simulink model "s_heli3d_fuzzy"  (R2023a)
settings: Solver=ode1  StartTime=0.0  StopTime=60  FixedStep=0.002  RelTol=1e-3  EnableMultiTasking=on
values from neighbouring files (symbols this model uses):
  A = sys.A    [read_model.m]
  B = sys.B    [read_model.m]
  CMD_RATE_LIMIT = 45.0 * pi / 180    (= 0.785398163397)    [setup_lab_heli_3d.m]
  K_AMP = 3    [setup_lab_heli_3d.m]
  VMAX_AMP = 24    [setup_lab_heli_3d.m]
  VMAX_DAC = 10    [setup_lab_heli_3d.m]
libraries: simulink_extras x6, statsLibrary x4
settings Model: ExtModeTrigDuration=5000  Creator=MLevis  LastModifiedBy=hackbrian
settings SolverCC: AlgebraicLoopSolver=TrustRegion  PositivePriorityOrder=on
settings DataIOCC: LimitDataPoints=on  SaveFormat=Array  SignalLoggingSaveFormat=ModelDataLogs  ReturnWorkspaceOutputs=off
settings OptimizationCC: BooleanDataType=off  OptimizeBlockIOStorage=off  BufferReuse=off  ExpressionFolding=off  ExpressionDepthLimit=2147483647  LocalBlockOutputs=off  InitFltsAndDblsToZero=on  LifeSpan=inf
settings DebuggingCC: SaveWithParameterizedLinksMsg=none  UnderspecifiedInitializationDetection=Classic  MergeDetectMultiDrivingBlocksExec=none  SignalResolutionControl=TryResolveAllWithWarning  SolverPrmCheckMsg=warning  MultiTaskDSMMsg=warning  MultiTaskCondExecSysMsg=none  FcnCallInpInsideContextMsg=warning  UnconnectedInputMsg=warning  UnconnectedOutputMsg=warning  UnconnectedLineMsg=warning  StateNameClashWarn=warning  SFUnexpectedBacktrackingDiag=warning  SFNoUnconditionalDefaultTransitionDiag=warning  SFExecutionAtInitializationDiag=none  ArithmeticOperatorsInVariantConditions=warning
settings HardwareCC: ProdBitPerPointer=32  ProdBitPerSizeT=32  ProdBitPerPtrDiffT=32  ProdLargestAtomicFloat=None  ProdIntDivRoundTo=Undefined  ProdEndianess=Unspecified  ProdWordSize=32  ProdHWDeviceType=32-bit Generic
settings ModelReferenceCC: PropagateSignalLabelsOutOfModel=off
settings RTWCC: Description=QUARC Win32 Target  SystemTargetFile=quarc_windows.tlc  TemplateMakefile=quarc_default_tmf
settings CodeAppCC: StateflowObjectComments=on
settings STFCustomTargetCC: TargetFcnLib=ansi_tfl_tmw.mat  TargetPreCompLibLocation=C:\DOCUME~1\ALLUSE~1\APPLIC~1\QUARC\lib\2007a\windows\release  TargetLangStandard=C89/C90 (ANSI)  ConcurrentExecutionCompliant=off  CPPClassGenCompliant=on  UseToolchainInfoCompliant=off  SystemTargetFile=quarc_windows.tlc
settings GRTTargetCC: TargetFcnLib=ansi_tfl_tmw.mat  TargetPreCompLibLocation=C:\DOCUME~1\ALLUSE~1\APPLIC~1\QUARC\lib\2007a\windows\release  TargetLangStandard=C89/C90 (ANSI)  ParMdlRefBuildCompliant=off  CompOptLevelCompliant=off  ConcurrentExecutionCompliant=off  CombineOutputUpdateFcns=off  MatFileLogging=off  GRTInterface=on  UseToolchainInfoCompliant=off  ExtMode=on  ExtModeMexFile=quarc_comm
settings ConfigComp: CovMetricSettings=dw  CovSaveCumulativeToWorkspaceVar=on  CovSaveSingleToWorkspaceVar=on

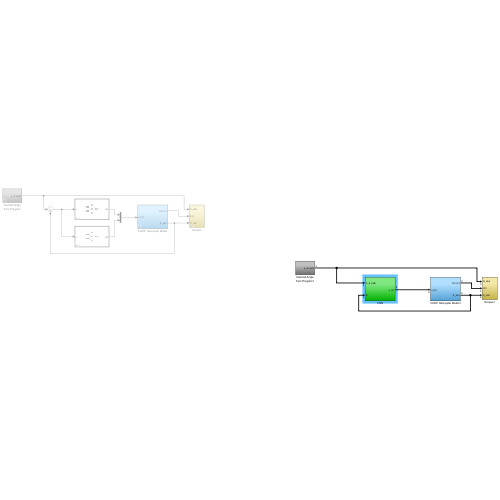
[thumbnail: Simulink's stored preview of the top-level diagram]
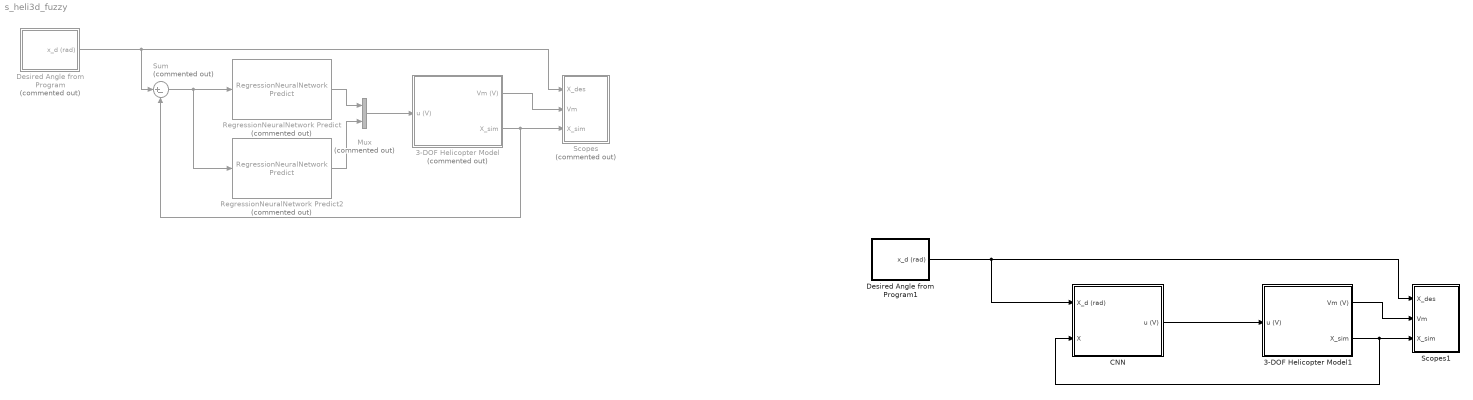
== system s_heli3d_fuzzy ==
  3-DOF Helicopter Model : Subsystem  Commented=on
  3-DOF Helicopter Model1 : Subsystem
  CNN : Subsystem  AncestorBlock=heli_2d_lib/2DOF HELI: FF+LQR+I Controller
      settings: LibrarySourceBlock=|
      | heli_2d_lib/2DOF HELI:
      | FF+LQR+I Controller
  Desired Angle from Program : Subsystem  Commented=on
  Desired Angle from Program1 : Subsystem
  Mux : Mux  Commented=on  Inputs=2
  RegressionNeuralNetwork Predict : statsLibrary/Regression/RegressionNeuralNetwork Predict  Commented=on  TrainedLearner=Mdl_voltage1  OutMin=[]  OutMax=[]  OutputLayerOutMin=[]  OutputLayerOutMax=[]  OutputLayerAdditionOutMin=[]  OutputLayerAdditionOutMax=[]  LayerSelector=Layer 1  Layer1OutMin=[]  Layer1OutMax=[]  Layer1AdditionOutMin=[]  Layer1AdditionOutMax=[]  Layer2OutMin=[]  Layer2OutMax=[]  Layer2AdditionOutMin=[]  Layer2AdditionOutMax=[]  Layer3OutMin=[]  Layer3OutMax=[]  Layer3AdditionOutMin=[]  Layer3AdditionOutMax=[]  Layer4OutMin=[]  Layer4OutMax=[]  Layer4AdditionOutMin=[]  Layer4AdditionOutMax=[]  Layer5OutMin=[]  Layer5OutMax=[]  Layer5AdditionOutMin=[]  Layer5AdditionOutMax=[]  Layer6OutMin=[]  Layer6OutMax=[]  Layer6AdditionOutMin=[]  Layer6AdditionOutMax=[]  Layer7OutMin=[]  Layer7OutMax=[]  Layer7AdditionOutMin=[]  Layer7AdditionOutMax=[]  Layer8OutMin=[]  Layer8OutMax=[]  Layer8AdditionOutMin=[]  Layer8AdditionOutMax=[]  Layer9OutMin=[]  Layer9OutMax=[]  Layer9AdditionOutMin=[]  Layer9AdditionOutMax=[]  Layer10OutMin=[]  Layer10OutMax=[]  Layer10AdditionOutMin=[]  Layer10AdditionOutMax=[]  Layer11OutMin=[]  Layer11OutMax=[]  Layer11AdditionOutMin=[]  Layer11AdditionOutMax=[]  StandardizedInputOutMin=[]  StandardizedInputOutMax=[]  NumHiddenLayers=1
  RegressionNeuralNetwork Predict2 : statsLibrary/Regression/RegressionNeuralNetwork Predict  Commented=on  TrainedLearner=Mdl_voltage2  OutMin=[]  OutMax=[]  OutputLayerOutMin=[]  OutputLayerOutMax=[]  OutputLayerAdditionOutMin=[]  OutputLayerAdditionOutMax=[]  LayerSelector=Layer 1  Layer1OutMin=[]  Layer1OutMax=[]  Layer1AdditionOutMin=[]  Layer1AdditionOutMax=[]  Layer2OutMin=[]  Layer2OutMax=[]  Layer2AdditionOutMin=[]  Layer2AdditionOutMax=[]  Layer3OutMin=[]  Layer3OutMax=[]  Layer3AdditionOutMin=[]  Layer3AdditionOutMax=[]  Layer4OutMin=[]  Layer4OutMax=[]  Layer4AdditionOutMin=[]  Layer4AdditionOutMax=[]  Layer5OutMin=[]  Layer5OutMax=[]  Layer5AdditionOutMin=[]  Layer5AdditionOutMax=[]  Layer6OutMin=[]  Layer6OutMax=[]  Layer6AdditionOutMin=[]  Layer6AdditionOutMax=[]  Layer7OutMin=[]  Layer7OutMax=[]  Layer7AdditionOutMin=[]  Layer7AdditionOutMax=[]  Layer8OutMin=[]  Layer8OutMax=[]  Layer8AdditionOutMin=[]  Layer8AdditionOutMax=[]  Layer9OutMin=[]  Layer9OutMax=[]  Layer9AdditionOutMin=[]  Layer9AdditionOutMax=[]  Layer10OutMin=[]  Layer10OutMax=[]  Layer10AdditionOutMin=[]  Layer10AdditionOutMax=[]  Layer11OutMin=[]  Layer11OutMax=[]  Layer11AdditionOutMin=[]  Layer11AdditionOutMax=[]  StandardizedInputOutMin=[]  StandardizedInputOutMax=[]  NumHiddenLayers=1
  Scopes : Subsystem  Commented=on
  Scopes1 : Subsystem
  Sum : Sum  Commented=on  Inputs=|+-
  wires:
  Desired Angle from Program/1(x_d (rad)) -> Sum/1, Scopes/1(X_des)
  3-DOF Helicopter Model/2(X_sim) -> Scopes/3(X_sim), Sum/2
  3-DOF Helicopter Model/1(Vm (V)) -> Scopes/2(Vm)
  Sum/1 -> RegressionNeuralNetwork Predict/1, RegressionNeuralNetwork Predict2/1
  Mux/1 -> 3-DOF Helicopter Model/1(u (V))
  RegressionNeuralNetwork Predict/1 -> Mux/1
  RegressionNeuralNetwork Predict2/1 -> Mux/2
  3-DOF Helicopter Model1/2(X_sim) -> CNN/2(X), Scopes1/3(X_sim)
  Desired Angle from Program1/1(x_d (rad)) -> CNN/1(X_d (rad)), Scopes1/1(X_des)
  3-DOF Helicopter Model1/1(Vm (V)) -> Scopes1/2(Vm)
  CNN/1(u (V)) -> 3-DOF Helicopter Model1/1(u (V))

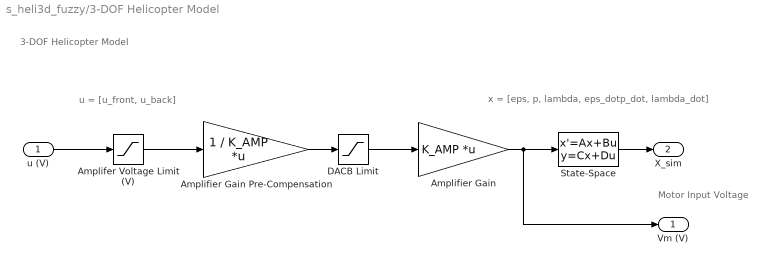
== system s_heli3d_fuzzy/3-DOF Helicopter Model ==
  note: x = [eps, p, lambda, eps_dotp_dot, lambda_dot]
  note: u = [u_front, u_back]
  note: Motor Input Voltage
  note: 3-DOF Helicopter Model
  u (V) : Inport
  Amplifer Voltage Limit (V) : Saturate  UpperLimit=VMAX_AMP  LowerLimit=-VMAX_AMP
  Amplifier Gain : Gain  Gain=K_AMP  Multiplication=Matrix(K*u)  SaturateOnIntegerOverflow=on  OutDataTypeStr=Inherit: Same as input  ParamDataTypeStr=Inherit: Same as input
  Amplifier Gain Pre-Compensation : Gain  Gain=1 / K_AMP  Multiplication=Matrix(K*u)  SaturateOnIntegerOverflow=on  OutDataTypeStr=Inherit: Same as input  ParamDataTypeStr=Inherit: Same as input
  DACB Limit : Saturate  UpperLimit=VMAX_DAC  LowerLimit=-VMAX_DAC
  State-Space : StateSpace  A=A  B=B  C=eye(6,6)  D=zeros(6,2)  InitialCondition=0
  Vm (V) : Outport
  X_sim : Outport  Port=2
  wires:
  u (V)/1 -> Amplifer Voltage Limit (V)/1
  Amplifier Gain/1 -> Vm (V)/1, State-Space/1
  State-Space/1 -> X_sim/1
  Amplifer Voltage Limit (V)/1 -> Amplifier Gain Pre-Compensation/1
  Amplifier Gain Pre-Compensation/1 -> DACB Limit/1
  DACB Limit/1 -> Amplifier Gain/1

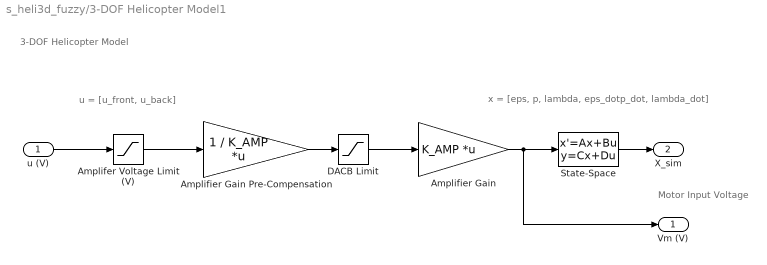
== system s_heli3d_fuzzy/3-DOF Helicopter Model1 ==
  note: x = [eps, p, lambda, eps_dotp_dot, lambda_dot]
  note: u = [u_front, u_back]
  note: Motor Input Voltage
  note: 3-DOF Helicopter Model
  u (V) : Inport
  Amplifer Voltage Limit (V) : Saturate  UpperLimit=VMAX_AMP  LowerLimit=-VMAX_AMP
  Amplifier Gain : Gain  Gain=K_AMP  Multiplication=Matrix(K*u)  SaturateOnIntegerOverflow=on  OutDataTypeStr=Inherit: Same as input  ParamDataTypeStr=Inherit: Same as input
  Amplifier Gain Pre-Compensation : Gain  Gain=1 / K_AMP  Multiplication=Matrix(K*u)  SaturateOnIntegerOverflow=on  OutDataTypeStr=Inherit: Same as input  ParamDataTypeStr=Inherit: Same as input
  DACB Limit : Saturate  UpperLimit=VMAX_DAC  LowerLimit=-VMAX_DAC
  State-Space : StateSpace  A=A  B=B  C=eye(6,6)  D=zeros(6,2)  InitialCondition=0
  Vm (V) : Outport
  X_sim : Outport  Port=2
  wires:
  u (V)/1 -> Amplifer Voltage Limit (V)/1
  Amplifier Gain/1 -> Vm (V)/1, State-Space/1
  State-Space/1 -> X_sim/1
  Amplifer Voltage Limit (V)/1 -> Amplifier Gain Pre-Compensation/1
  Amplifier Gain Pre-Compensation/1 -> DACB Limit/1
  DACB Limit/1 -> Amplifier Gain/1

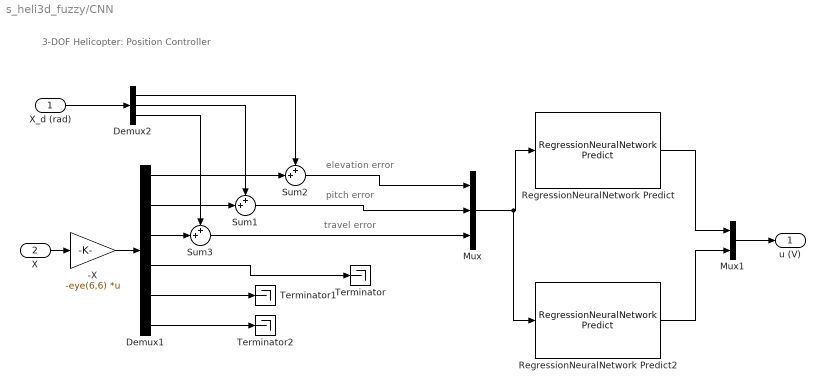
== system s_heli3d_fuzzy/CNN ==
  note: elevation error
  note: pitch error
  note: 3-DOF Helicopter: Position Controller
  note: travel error
  X_d (rad) : Inport
  X : Inport  Port=2
  -X : Gain  Gain=-eye(6,6)  Multiplication=Matrix(K*u)
  Demux1 : Demux  Outputs=6
  Demux2 : Demux  Outputs=3
  Mux : Mux  Inputs=3
  Mux1 : Mux  Inputs=2
  RegressionNeuralNetwork Predict : statsLibrary/Regression/RegressionNeuralNetwork Predict  TrainedLearner=Mdl_voltage1  OutMin=[]  OutMax=[]  OutputLayerOutMin=[]  OutputLayerOutMax=[]  OutputLayerAdditionOutMin=[]  OutputLayerAdditionOutMax=[]  LayerSelector=Layer 1  Layer1OutMin=[]  Layer1OutMax=[]  Layer1AdditionOutMin=[]  Layer1AdditionOutMax=[]  Layer2OutMin=[]  Layer2OutMax=[]  Layer2AdditionOutMin=[]  Layer2AdditionOutMax=[]  Layer3OutMin=[]  Layer3OutMax=[]  Layer3AdditionOutMin=[]  Layer3AdditionOutMax=[]  Layer4OutMin=[]  Layer4OutMax=[]  Layer4AdditionOutMin=[]  Layer4AdditionOutMax=[]  Layer5OutMin=[]  Layer5OutMax=[]  Layer5AdditionOutMin=[]  Layer5AdditionOutMax=[]  Layer6OutMin=[]  Layer6OutMax=[]  Layer6AdditionOutMin=[]  Layer6AdditionOutMax=[]  Layer7OutMin=[]  Layer7OutMax=[]  Layer7AdditionOutMin=[]  Layer7AdditionOutMax=[]  Layer8OutMin=[]  Layer8OutMax=[]  Layer8AdditionOutMin=[]  Layer8AdditionOutMax=[]  Layer9OutMin=[]  Layer9OutMax=[]  Layer9AdditionOutMin=[]  Layer9AdditionOutMax=[]  Layer10OutMin=[]  Layer10OutMax=[]  Layer10AdditionOutMin=[]  Layer10AdditionOutMax=[]  Layer11OutMin=[]  Layer11OutMax=[]  Layer11AdditionOutMin=[]  Layer11AdditionOutMax=[]  StandardizedInputOutMin=[]  StandardizedInputOutMax=[]  NumHiddenLayers=1
  RegressionNeuralNetwork Predict2 : statsLibrary/Regression/RegressionNeuralNetwork Predict  TrainedLearner=Mdl_voltage2  OutMin=[]  OutMax=[]  OutputLayerOutMin=[]  OutputLayerOutMax=[]  OutputLayerAdditionOutMin=[]  OutputLayerAdditionOutMax=[]  LayerSelector=Layer 1  Layer1OutMin=[]  Layer1OutMax=[]  Layer1AdditionOutMin=[]  Layer1AdditionOutMax=[]  Layer2OutMin=[]  Layer2OutMax=[]  Layer2AdditionOutMin=[]  Layer2AdditionOutMax=[]  Layer3OutMin=[]  Layer3OutMax=[]  Layer3AdditionOutMin=[]  Layer3AdditionOutMax=[]  Layer4OutMin=[]  Layer4OutMax=[]  Layer4AdditionOutMin=[]  Layer4AdditionOutMax=[]  Layer5OutMin=[]  Layer5OutMax=[]  Layer5AdditionOutMin=[]  Layer5AdditionOutMax=[]  Layer6OutMin=[]  Layer6OutMax=[]  Layer6AdditionOutMin=[]  Layer6AdditionOutMax=[]  Layer7OutMin=[]  Layer7OutMax=[]  Layer7AdditionOutMin=[]  Layer7AdditionOutMax=[]  Layer8OutMin=[]  Layer8OutMax=[]  Layer8AdditionOutMin=[]  Layer8AdditionOutMax=[]  Layer9OutMin=[]  Layer9OutMax=[]  Layer9AdditionOutMin=[]  Layer9AdditionOutMax=[]  Layer10OutMin=[]  Layer10OutMax=[]  Layer10AdditionOutMin=[]  Layer10AdditionOutMax=[]  Layer11OutMin=[]  Layer11OutMax=[]  Layer11AdditionOutMin=[]  Layer11AdditionOutMax=[]  StandardizedInputOutMin=[]  StandardizedInputOutMax=[]  NumHiddenLayers=1
  Sum1 : Sum  Inputs=++|
  Sum2 : Sum  Inputs=++|
  Sum3 : Sum  Inputs=++|
  Terminator : Terminator
  Terminator1 : Terminator
  Terminator2 : Terminator
  u (V) : Outport
  wires:
  Demux1/2 -> Sum1/2
  Demux2/2 -> Sum1/1
  Demux2/1 -> Sum2/1
  X_d (rad)/1 -> Demux2/1
  Demux1/1 -> Sum2/2
  X/1 -> -X/1
  Sum1/1 -> Mux/2
  -X/1 -> Demux1/1
  Demux2/3 -> Sum3/1
  Demux1/3 -> Sum3/2
  Sum3/1 -> Mux/3
  Mux1/1 -> u (V)/1
  RegressionNeuralNetwork Predict/1 -> Mux1/1
  RegressionNeuralNetwork Predict2/1 -> Mux1/2
  Demux1/4 -> Terminator/1
  Demux1/5 -> Terminator1/1
  Demux1/6 -> Terminator2/1
  Sum2/1 -> Mux/1
  Mux/1 -> RegressionNeuralNetwork Predict2/1, RegressionNeuralNetwork Predict/1

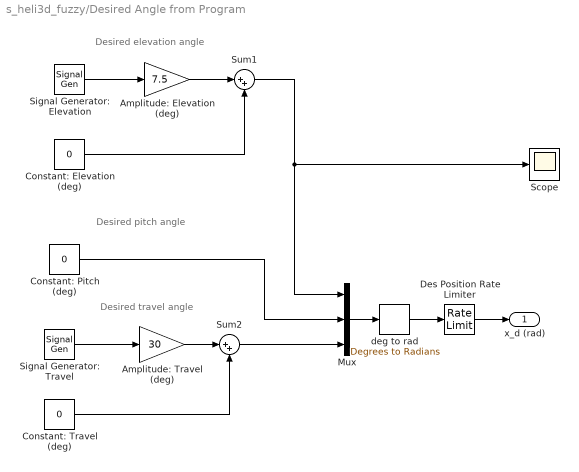
== system s_heli3d_fuzzy/Desired Angle from Program ==
  note: Desired elevation angle
  note: Desired travel angle
  note: Desired pitch angle
  Amplitude: Elevation (deg) : Gain  Gain=7.5
  Amplitude: Travel (deg) : Gain  Gain=30
  Constant: Elevation (deg) : Constant  Value=0
  Constant: Pitch (deg) : Constant  Value=0
  Constant: Travel (deg) : Constant  Value=0
  Des Position Rate Limiter : RateLimiter  RisingSlewLimit=CMD_RATE_LIMIT  FallingSlewLimit=-CMD_RATE_LIMIT  SampleTimeMode=inherited
  Mux : Mux  Inputs=3
  Scope : Scope
  Signal Generator: Elevation : SignalGenerator  WaveForm=square  Frequency=0.04
  Signal Generator: Travel : SignalGenerator  WaveForm=square  Frequency=0.03
  Sum1 : Sum  Inputs=|++
  Sum2 : Sum  Inputs=|++
  deg to rad : simulink_extras/Transformations/Degrees to Radians
  x_d (rad) : Outport
  wires:
  Mux/1 -> deg to rad/1
  Constant: Elevation (deg)/1 -> Sum1/2
  Amplitude: Elevation (deg)/1 -> Sum1/1
  Signal Generator: Elevation/1 -> Amplitude: Elevation (deg)/1
  Constant: Travel (deg)/1 -> Sum2/2
  Amplitude: Travel (deg)/1 -> Sum2/1
  Signal Generator: Travel/1 -> Amplitude: Travel (deg)/1
  Sum2/1 -> Mux/3
  deg to rad/1 -> Des Position Rate Limiter/1
  Constant: Pitch (deg)/1 -> Mux/2
  Sum1/1 -> Mux/1, Scope/1
  Des Position Rate Limiter/1 -> x_d (rad)/1

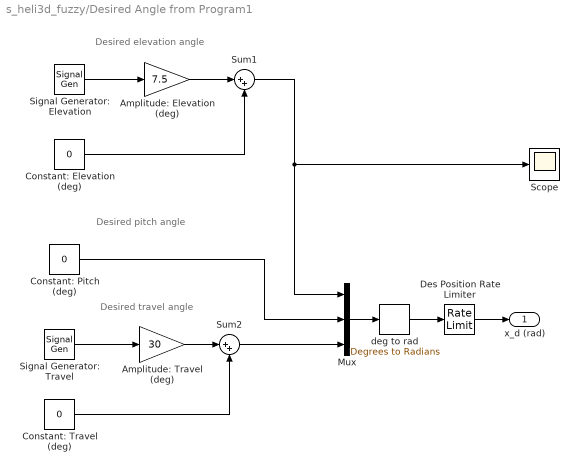
== system s_heli3d_fuzzy/Desired Angle from Program1 ==
  note: Desired elevation angle
  note: Desired travel angle
  note: Desired pitch angle
  Amplitude: Elevation (deg) : Gain  Gain=7.5
  Amplitude: Travel (deg) : Gain  Gain=30
  Constant: Elevation (deg) : Constant  Value=0
  Constant: Pitch (deg) : Constant  Value=0
  Constant: Travel (deg) : Constant  Value=0
  Des Position Rate Limiter : RateLimiter  RisingSlewLimit=CMD_RATE_LIMIT  FallingSlewLimit=-CMD_RATE_LIMIT  SampleTimeMode=inherited
  Mux : Mux  Inputs=3
  Scope : Scope
  Signal Generator: Elevation : SignalGenerator  WaveForm=square  Frequency=0.04
  Signal Generator: Travel : SignalGenerator  WaveForm=square  Frequency=0.03
  Sum1 : Sum  Inputs=|++
  Sum2 : Sum  Inputs=|++
  deg to rad : simulink_extras/Transformations/Degrees to Radians
  x_d (rad) : Outport
  wires:
  Mux/1 -> deg to rad/1
  Constant: Elevation (deg)/1 -> Sum1/2
  Amplitude: Elevation (deg)/1 -> Sum1/1
  Signal Generator: Elevation/1 -> Amplitude: Elevation (deg)/1
  Constant: Travel (deg)/1 -> Sum2/2
  Amplitude: Travel (deg)/1 -> Sum2/1
  Signal Generator: Travel/1 -> Amplitude: Travel (deg)/1
  Sum2/1 -> Mux/3
  deg to rad/1 -> Des Position Rate Limiter/1
  Constant: Pitch (deg)/1 -> Mux/2
  Sum1/1 -> Mux/1, Scope/1
  Des Position Rate Limiter/1 -> x_d (rad)/1

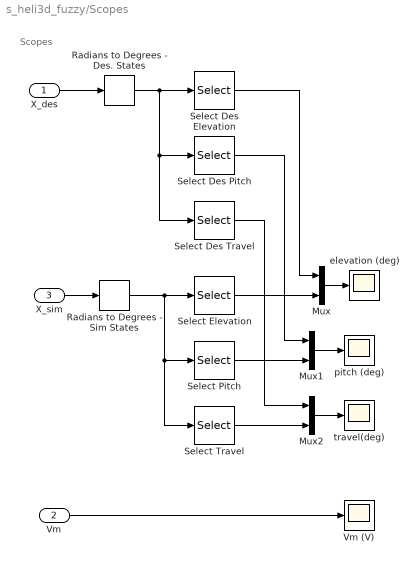
== system s_heli3d_fuzzy/Scopes ==
  note: Scopes
  X_des : Inport
  Vm : Inport  Port=2
  X_sim : Inport  Port=3
  Mux : Mux  Inputs=2
  Mux1 : Mux  Inputs=2
  Mux2 : Mux  Inputs=2
  Radians to Degrees - Des. States : simulink_extras/Transformations/Radians to Degrees
  Radians to Degrees - Sim States : simulink_extras/Transformations/Radians to Degrees
  Select Des Elevation : Selector  InputPortWidth=3  IndexOptions=Index vector (dialog)  Indices=1  OutputSizes=1
  Select Des Pitch : Selector  InputPortWidth=3  IndexOptions=Index vector (dialog)  Indices=2  OutputSizes=1
  Select Des Travel : Selector  InputPortWidth=3  IndexOptions=Index vector (dialog)  Indices=3  OutputSizes=1
  Select Elevation : Selector  InputPortWidth=6  IndexOptions=Index vector (dialog)  Indices=1  OutputSizes=1
  Select Pitch : Selector  InputPortWidth=6  IndexOptions=Index vector (dialog)  Indices=2  OutputSizes=1
  Select Travel : Selector  InputPortWidth=6  IndexOptions=Index vector (dialog)  Indices=3  OutputSizes=1
  Vm (V) : Scope
  elevation (deg) : Scope
  pitch (deg) : Scope
  travel(deg) : Scope
  wires:
  X_des/1 -> Radians to Degrees - Des. States/1
  X_sim/1 -> Radians to Degrees - Sim States/1
  Mux/1 -> elevation (deg)/1
  Mux1/1 -> pitch (deg)/1
  Vm/1 -> Vm (V)/1
  Radians to Degrees - Sim States/1 -> Select Elevation/1, Select Pitch/1, Select Travel/1
  Mux2/1 -> travel(deg)/1
  Select Elevation/1 -> Mux/2
  Select Pitch/1 -> Mux1/2
  Select Travel/1 -> Mux2/2
  Radians to Degrees - Des. States/1 -> Select Des Elevation/1, Select Des Pitch/1, Select Des Travel/1
  Select Des Elevation/1 -> Mux/1
  Select Des Pitch/1 -> Mux1/1
  Select Des Travel/1 -> Mux2/1

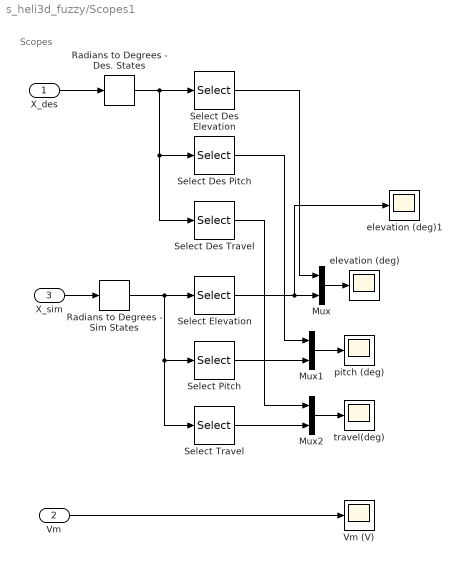
== system s_heli3d_fuzzy/Scopes1 ==
  note: Scopes
  X_des : Inport
  Vm : Inport  Port=2
  X_sim : Inport  Port=3
  Mux : Mux  Inputs=2
  Mux1 : Mux  Inputs=2
  Mux2 : Mux  Inputs=2
  Radians to Degrees - Des. States : simulink_extras/Transformations/Radians to Degrees
  Radians to Degrees - Sim States : simulink_extras/Transformations/Radians to Degrees
  Select Des Elevation : Selector  InputPortWidth=3  IndexOptions=Index vector (dialog)  Indices=1  OutputSizes=1
  Select Des Pitch : Selector  InputPortWidth=3  IndexOptions=Index vector (dialog)  Indices=2  OutputSizes=1
  Select Des Travel : Selector  InputPortWidth=3  IndexOptions=Index vector (dialog)  Indices=3  OutputSizes=1
  Select Elevation : Selector  InputPortWidth=6  IndexOptions=Index vector (dialog)  Indices=1  OutputSizes=1
  Select Pitch : Selector  InputPortWidth=6  IndexOptions=Index vector (dialog)  Indices=2  OutputSizes=1
  Select Travel : Selector  InputPortWidth=6  IndexOptions=Index vector (dialog)  Indices=3  OutputSizes=1
  Vm (V) : Scope
  elevation (deg) : Scope
  elevation (deg)1 : Scope
  pitch (deg) : Scope
  travel(deg) : Scope
  wires:
  X_des/1 -> Radians to Degrees - Des. States/1
  X_sim/1 -> Radians to Degrees - Sim States/1
  Mux/1 -> elevation (deg)/1
  Mux1/1 -> pitch (deg)/1
  Vm/1 -> Vm (V)/1
  Radians to Degrees - Sim States/1 -> Select Elevation/1, Select Pitch/1, Select Travel/1
  Mux2/1 -> travel(deg)/1
  Select Elevation/1 -> elevation (deg)1/1, Mux/2
  Select Pitch/1 -> Mux1/2
  Select Travel/1 -> Mux2/2
  Radians to Degrees - Des. States/1 -> Select Des Elevation/1, Select Des Pitch/1, Select Des Travel/1
  Select Des Elevation/1 -> Mux/1
  Select Des Pitch/1 -> Mux1/1
  Select Des Travel/1 -> Mux2/1
